simulink library "hostCommsLib"  (R2014b)
settings: Solver=ode45  StartTime=0.0  StopTime=10.0  RelTol=1e-3
undefined symbols (not defined in the file): RobotID
settings Model: Creator=ksurende  LastModifiedBy=ksurende

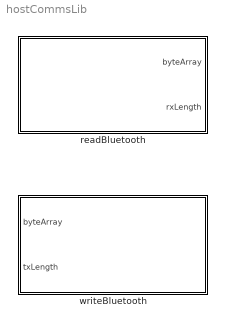
== system hostCommsLib ==
  readBluetooth : MATLAB Function  TreatAsAtomicUnit=on  mask{robotId=RobotID.NXT_BEN, numBytes=0}
      mask help: Robot Bluetooth Read
  writeBluetooth : MATLAB Function  TreatAsAtomicUnit=on  mask{robotId=RobotID.NXT_BEN}
      mask help: Robot Bluetooth Write

== matlab function hostCommsLib/writeBluetooth ==
  data: robotId parameter Enum: RobotID; byteArray input uint8; txLength input double
function writeBluetooth(robotId,byteArray,txLength)
%#codegen

coder.extrinsic('comms.writeWrapper');
comms.writeWrapper(robotId,uint8(byteArray),uint8(txLength));

== matlab function hostCommsLib/readBluetooth ==
  data: robotId parameter Enum: RobotID; numBytes parameter uint8; byteArray output uint8; rxLength output double
function [byteArray,rxLength] = readBluetooth(robotId,numBytes)
%#codegen

coder.extrinsic('comms.readWrapper')

byteArray = zeros([1,numBytes],'uint8');
rxLength = 0;
[byteArray,rxLength] = comms.readWrapper(robotId,uint8(numBytes));
